simulink model "foc"  (R2022b)
settings: Solver=VariableStepAuto  StartTime=0.0  StopTime=1  RelTol=1e-3
libraries: simulink x1
settings Model: Creator=15403  LastModifiedBy=15403

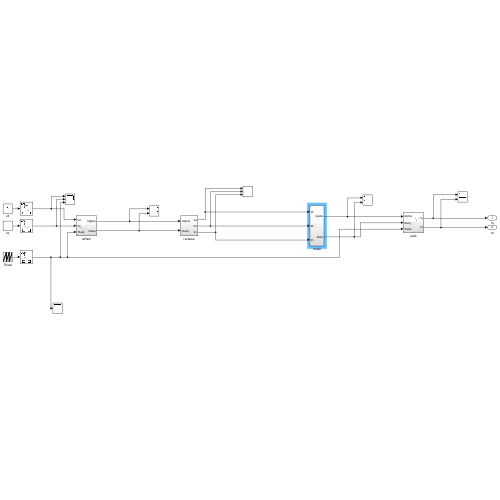
[thumbnail: Simulink's stored preview of the top-level diagram]
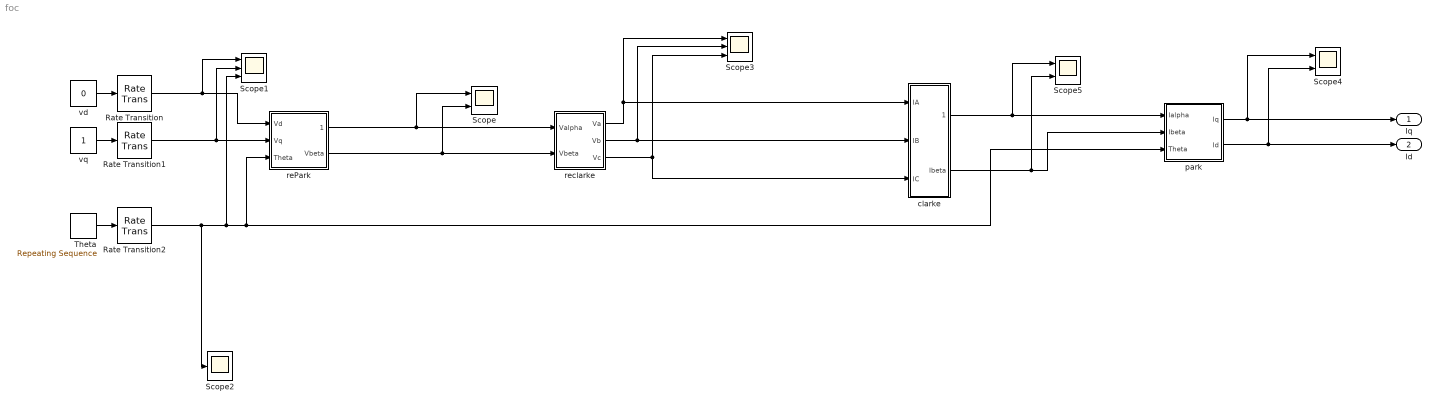
== system foc ==
  Rate Transition : RateTransition
  Rate Transition1 : RateTransition
  Rate Transition2 : RateTransition
  Scope : Scope  NumInputPorts=2
  Scope1 : Scope  NumInputPorts=3
  Scope2 : Scope
  Scope3 : Scope  NumInputPorts=3
  Scope4 : Scope  NumInputPorts=2
  Scope5 : Scope  NumInputPorts=2
  Theta : simulink/Sources/Repeating Sequence  rep_seq_t=[0 0.1]  rep_seq_y=[0 360]
  clarke : Subsystem
  park : Subsystem
  rePark : Subsystem
  reclarke : Subsystem
  vd : Constant  Value=0
  vq : Constant
  Iq : Outport
  Id : Outport  Port=2
  wires:
  Rate Transition/1 -> Scope1/1, rePark/1(Vd)
  Theta/1 -> Rate Transition2/1
  rePark/2(Vbeta) -> reclarke/2(Vbeta), Scope/2
  Rate Transition2/1 -> Scope2/1, park/3(Theta), rePark/3(Theta), Scope1/3
  vq/1 -> Rate Transition1/1
  vd/1 -> Rate Transition/1
  Rate Transition1/1 -> Scope1/2, rePark/2(Vq)
  rePark/1(Valpha) -> reclarke/1(Valpha), Scope/1
  reclarke/1(Va) -> Scope3/1, clarke/1(IA)
  reclarke/2(Vb) -> clarke/2(IB), Scope3/2
  reclarke/3(Vc) -> clarke/3(IC), Scope3/3
  clarke/2(Ibeta) -> Scope5/2, park/2(Ibeta)
  clarke/1(Ialpha) -> Scope5/1, park/1(Ialpha)
  park/1(Iq) -> Scope4/1, Iq/1
  park/2(Id) -> Scope4/2, Id/1

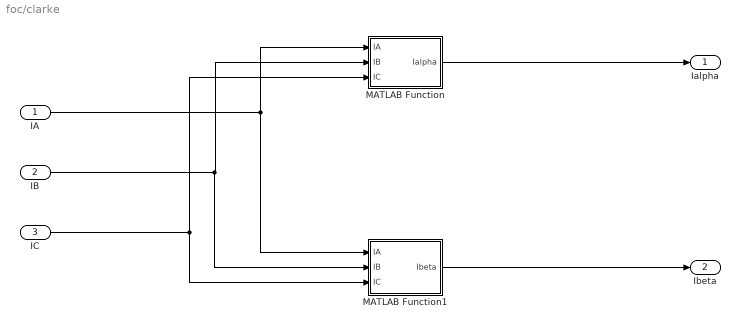
== system foc/clarke ==
  IA : Inport
  IB : Inport  Port=2
  IC : Inport  Port=3
  MATLAB Function : MATLAB Function  TreatAsAtomicUnit=on
  MATLAB Function1 : MATLAB Function  TreatAsAtomicUnit=on
  Ialpha : Outport
  Ibeta : Outport  Port=2
  wires:
  MATLAB Function1/1(Ibeta) -> Ibeta/1
  MATLAB Function/1(Ialpha) -> Ialpha/1
  IA/1 -> MATLAB Function1/1(IA), MATLAB Function/1(IA)
  IB/1 -> MATLAB Function1/2(IB), MATLAB Function/2(IB)
  IC/1 -> MATLAB Function/3(IC), MATLAB Function1/3(IC)

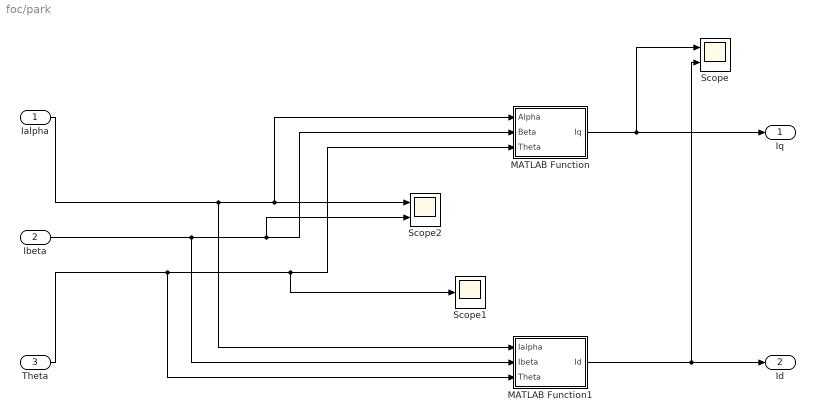
== system foc/park ==
  Ialpha : Inport
  Ibeta : Inport  Port=2
  Theta : Inport  Port=3
  MATLAB Function : MATLAB Function  TreatAsAtomicUnit=on
  MATLAB Function1 : MATLAB Function  TreatAsAtomicUnit=on
  Scope : Scope  NumInputPorts=2
  Scope1 : Scope
  Scope2 : Scope  NumInputPorts=2
  Iq : Outport
  Id : Outport  Port=2
  wires:
  MATLAB Function1/1(Id) -> Scope/2, Id/1
  Ialpha/1 -> MATLAB Function1/1(Ialpha), Scope2/1, MATLAB Function/1(Alpha)
  Ibeta/1 -> MATLAB Function1/2(Ibeta), Scope2/2, MATLAB Function/2(Beta)
  Theta/1 -> MATLAB Function1/3(Theta), Scope1/1, MATLAB Function/3(Theta)
  MATLAB Function/1(Iq) -> Iq/1, Scope/1

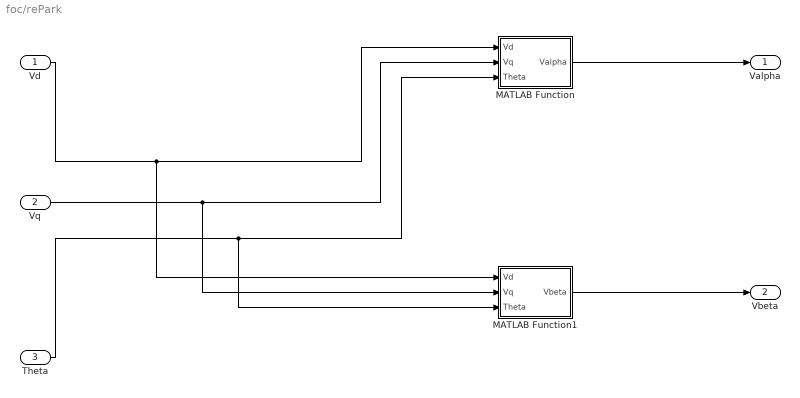
== system foc/rePark ==
  Vd : Inport
  Vq : Inport  Port=2
  Theta : Inport  Port=3
  MATLAB Function : MATLAB Function  TreatAsAtomicUnit=on
  MATLAB Function1 : MATLAB Function  TreatAsAtomicUnit=on
  Valpha : Outport
  Vbeta : Outport  Port=2
  wires:
  Theta/1 -> MATLAB Function1/3(Theta), MATLAB Function/3(Theta)
  MATLAB Function1/1(Vbeta) -> Vbeta/1
  Vq/1 -> MATLAB Function1/2(Vq), MATLAB Function/2(Vq)
  Vd/1 -> MATLAB Function1/1(Vd), MATLAB Function/1(Vd)
  MATLAB Function/1(Valpha) -> Valpha/1

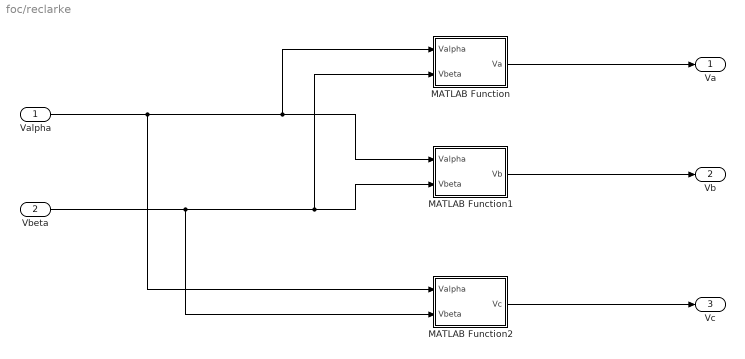
== system foc/reclarke ==
  Valpha : Inport
  Vbeta : Inport  Port=2
  MATLAB Function : MATLAB Function  TreatAsAtomicUnit=on
  MATLAB Function1 : MATLAB Function  TreatAsAtomicUnit=on
  MATLAB Function2 : MATLAB Function  TreatAsAtomicUnit=on
  Va : Outport
  Vb : Outport  Port=2
  Vc : Outport  Port=3
  wires:
  Valpha/1 -> MATLAB Function2/1(Valpha), MATLAB Function/1(Valpha), MATLAB Function1/1(Valpha)
  MATLAB Function1/1(Vb) -> Vb/1
  Vbeta/1 -> MATLAB Function2/2(Vbeta), MATLAB Function/2(Vbeta), MATLAB Function1/2(Vbeta)
  MATLAB Function/1(Va) -> Va/1
  MATLAB Function2/1(Vc) -> Vc/1

== matlab function foc/rePark/MATLAB Function1 ==
  data: Vd input; Vbeta output; Vq input; Theta input
function Vbeta = fcn(Vd, Vq, Theta)

Vbeta = Vq * cosd(Theta) + Vd * sind(Theta);

== matlab function foc/rePark/MATLAB Function ==
  data: Vd input; Valpha output; Vq input; Theta input
function Valpha = fcn(Vd, Vq, Theta)

Valpha = -Vq * sind(Theta) + Vd * cosd(Theta);

== matlab function foc/reclarke/MATLAB Function ==
  data: Valpha input; Va output; Vbeta input
function Va = fcn(Valpha, Vbeta)

Va = Valpha;

== matlab function foc/reclarke/MATLAB Function1 ==
  data: Valpha input; Vb output; Vbeta input
function Vb = fcn(Valpha, Vbeta)

Vb = -Valpha * sind(30) + Vbeta * cosd(30);

== matlab function foc/reclarke/MATLAB Function2 ==
  data: Valpha input; Vc output; Vbeta input
function Vc = fcn(Valpha, Vbeta)

Vc = -Valpha * sind(30) - Vbeta * cosd(30);

== matlab function foc/clarke/MATLAB Function ==
  data: Ialpha output; IA input; IB input; IC input
function Ialpha = fcn(IA, IB, IC)
%Ialpha = IA - (IB + IC) * cosd(60);
Ialpha = IA;

== matlab function foc/clarke/MATLAB Function1 ==
  data: IA input; Ibeta output; IB input; IC input
function Ibeta = fcn(IA, IB, IC)
Ibeta = 2/3 *(IB - IC) * cosd(30);
%Ibeta = (IA + 2*IB) / sqrt(3);

== matlab function foc/park/MATLAB Function ==
  data: Alpha input; Iq output; Beta input; Theta input
function Iq = fcn(Alpha, Beta, Theta)

Iq = -Alpha * sind(Theta) + Beta * cosd(Theta);

== matlab function foc/park/MATLAB Function1 ==
  data: Ialpha input; Id output; Ibeta input; Theta input
function Id = fcn(Ialpha, Ibeta, Theta)

Id = Ialpha * cosd(Theta) + Ibeta * sind(Theta);
